simulink model "differential_drive_kinematic_model"  (R2022b)
settings: Solver=VariableStepAuto  StartTime=0.0  StopTime=10.0  RelTol=1e-3
libraries: mobileRoboticsLib x2, robotmobilelib x1
settings Model: Creator=chris  LastModifiedBy=christian.badolo

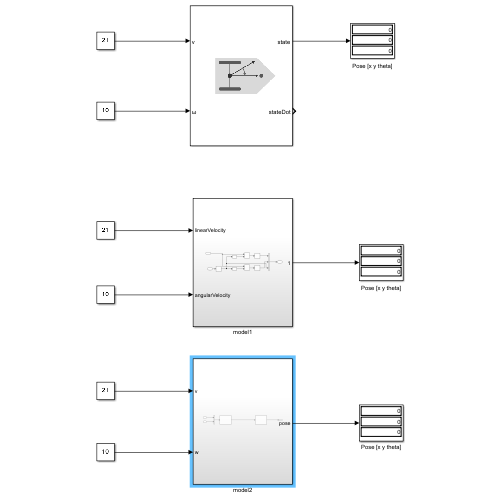
[thumbnail: Simulink's stored preview of the top-level diagram]
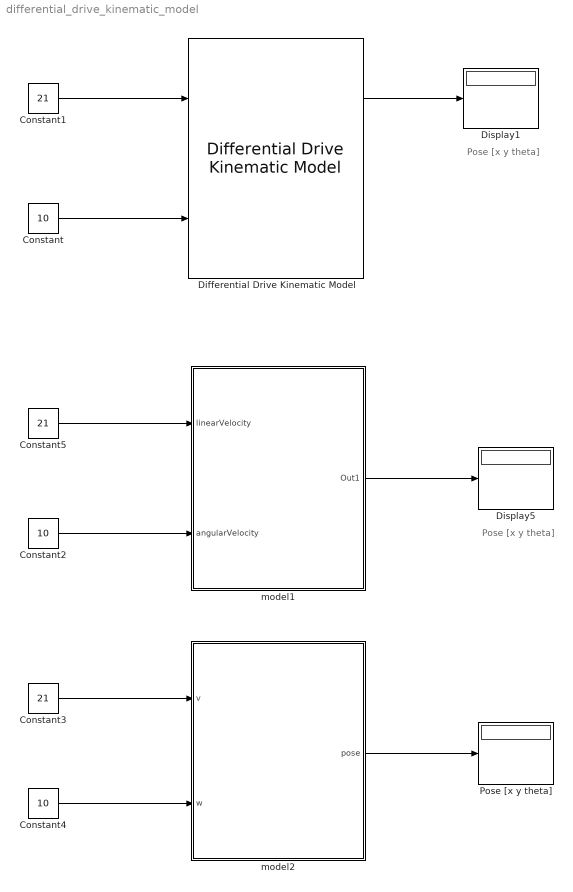
== system differential_drive_kinematic_model ==
  note: Pose [x y theta]
  note: Pose [x y theta]
  Constant : Constant  Value=10
  Constant1 : Constant  Value=21
  Constant2 : Constant  Value=10
  Constant3 : Constant  Value=21
  Constant4 : Constant  Value=10
  Constant5 : Constant  Value=21
  Differential Drive Kinematic Model : robotmobilelib/Differential Drive Kinematic Model  VehicleInputs=Vehicle Speed & Heading Angular Velocity  WheelRadius=0.05  WheelSpeedRange=[-inf inf]  TrackWidth=0.2  InitialState=[0; 0; 0]  SimulateUsing=Interpreted execution
  Display1 : Display
  Display5 : Display
  Pose [x y theta] : Display
  model1 : Subsystem
  model2 : Subsystem
  wires:
  Constant/1 -> Differential Drive Kinematic Model/2
  Constant1/1 -> Differential Drive Kinematic Model/1
  Differential Drive Kinematic Model/1 -> Display1/1
  model1/1(Out1) -> Display5/1
  Constant5/1 -> model1/1(linearVelocity)
  Constant2/1 -> model1/2(angularVelocity)
  Constant3/1 -> model2/1(v)
  Constant4/1 -> model2/2(w)
  model2/1(pose) -> Pose [x y theta]/1

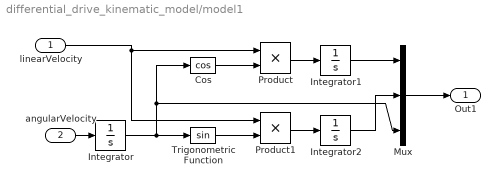
== system differential_drive_kinematic_model/model1 ==
  linearVelocity : Inport
  angularVelocity : Inport  Port=2
  Cos : Trigonometry  Operator=cos
  Integrator : Integrator
  Integrator1 : Integrator
  Integrator2 : Integrator
  Mux : Mux  Inputs=3
  Product : Product
  Product1 : Product
  Trigonometric Function : Trigonometry
  Out1 : Outport
  wires:
  Cos/1 -> Product/2
  Integrator/1 -> Cos/1, Mux/3, Trigonometric Function/1
  Product1/1 -> Integrator2/1
  Product/1 -> Integrator1/1
  Trigonometric Function/1 -> Product1/2
  angularVelocity/1 -> Integrator/1
  linearVelocity/1 -> Product1/1, Product/1
  Mux/1 -> Out1/1
  Integrator1/1 -> Mux/1
  Integrator2/1 -> Mux/2

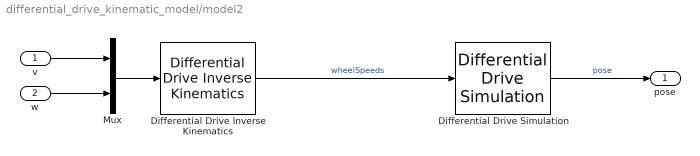
== system differential_drive_kinematic_model/model2 ==
  v : Inport
  w : Inport  Port=2
  Differential Drive Inverse Kinematics : mobileRoboticsLib/Kinematic Models/Differential Drive/Differential Drive Inverse Kinematics  wheelRadius=0.05  wheelBase=0.01
  Differential Drive Simulation : mobileRoboticsLib/Kinematic Models/Differential Drive/Differential Drive Simulation  wheelRadius=0.05  wheelBase=0.01  initX=0  initY=0  initAngle=0  Ts=-1
  Mux : Mux  Inputs=2
  pose : Outport
  wires:
  Mux/1 -> Differential Drive Inverse Kinematics/1
  Differential Drive Simulation/1 -> pose/1  "pose"
  Differential Drive Inverse Kinematics/1 -> Differential Drive Simulation/1  "wheelSpeeds"
  w/1 -> Mux/2
  v/1 -> Mux/1
